simulink subsystem "DCMotor"  (R2022b)
settings: Solver=VariableStepAuto  StartTime=0.0  StopTime=10.0  RelTol=1e-3
undefined symbols (not defined in the file): ProjectExample
settings Model: Creator=Ilya_Andriyanov  LastModifiedBy=user

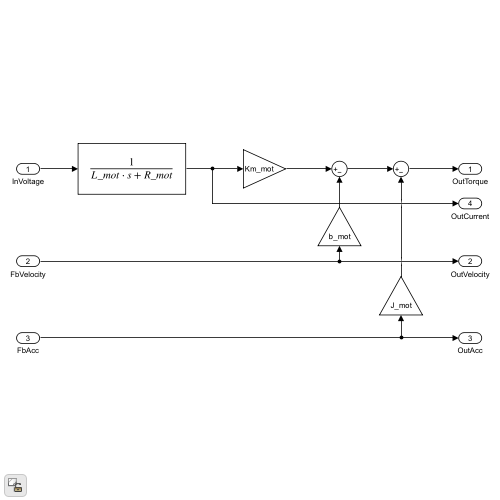
[thumbnail: Simulink's stored preview of the top-level diagram]
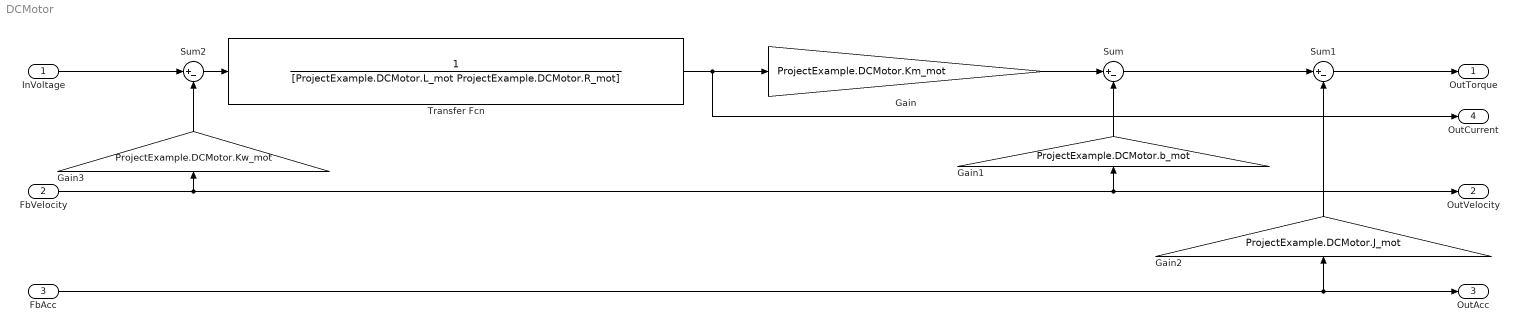
== system DCMotor ==
  InVoltage : Inport
  FbVelocity : Inport  Port=2
  FbAcc : Inport  Port=3
  Gain : Gain  Gain=ProjectExample.DCMotor.Km_mot
  Gain1 : Gain  Gain=ProjectExample.DCMotor.b_mot
  Gain2 : Gain  Gain=ProjectExample.DCMotor.J_mot
  Gain3 : Gain  Gain=ProjectExample.DCMotor.Kw_mot
  Sum : Sum  Inputs=|+-
  Sum1 : Sum  Inputs=|+-
  Sum2 : Sum  Inputs=|+-
  Transfer Fcn : TransferFcn  Denominator=[ProjectExample.DCMotor.L_mot ProjectExample.DCMotor.R_mot]
  OutTorque : Outport
  OutVelocity : Outport  Port=2
  OutAcc : Outport  Port=3
  OutCurrent : Outport  Port=4
  wires:
  FbVelocity/1 -> Gain3/1, Gain1/1, OutVelocity/1
  Transfer Fcn/1 -> Gain/1, OutCurrent/1
  Gain/1 -> Sum/1
  Sum/1 -> Sum1/1
  Sum1/1 -> OutTorque/1
  Gain1/1 -> Sum/2
  Gain2/1 -> Sum1/2
  FbAcc/1 -> Gain2/1, OutAcc/1
  Sum2/1 -> Transfer Fcn/1
  InVoltage/1 -> Sum2/1
  Gain3/1 -> Sum2/2
